simulink library "mech_stewart_control_deriv"  (Simulink 7.1)
values from neighbouring files (symbols this model uses):
  A = 100*freq    (= 314.159265359)    [mech_stewart_studies_setup.m]
libraries: mech_stewart_control_deriv x1
settings Model: Creator=batserve  LastModifiedBy=batserve  ExtModeAutoUpdateStatusClock=off

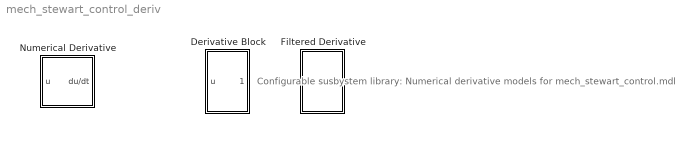
== system mech_stewart_control_deriv ==
  note: Configurable susbystem library:
      | Numerical derivative models for
      | mech_stewart_control.mdl
  Derivative Block : Subsystem
  Filtered Derivative : Subsystem
  "Numerical Derivative " : Subsystem  BlockChoice=Derivative Block
      settings: TemplateBlock=self  MemberBlocks=Derivative Block,Filtered Derivative

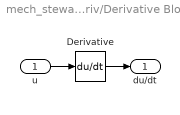
== system mech_stewart_control_deriv/Derivative Block ==
  u : Inport  OutDataType=sfix(16)  OutScaling=2^0
  Derivative : Derivative
  du/dt : Outport  OutDataType=sfix(16)  OutScaling=2^0
  wires:
  Derivative/1 -> du/dt/1
  u/1 -> Derivative/1

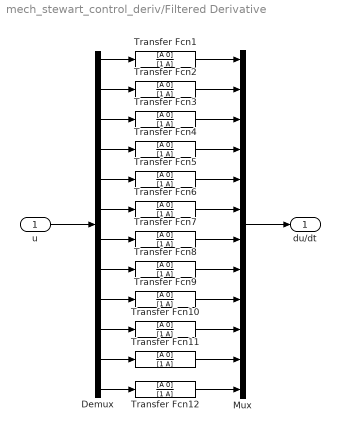
== system mech_stewart_control_deriv/Filtered Derivative ==
  u : Inport  OutDataType=sfix(16)  OutScaling=2^0
  Demux : Demux  Outputs=12
  Mux : Mux  Inputs=12
  Transfer Fcn{1..12} (12 alike) : TransferFcn  Numerator=[A 0]  Denominator=[1 A]
  du/dt : Outport  OutDataType=sfix(16)  OutScaling=2^0
  wires:
  Mux/1 -> du/dt/1
  u/1 -> Demux/1
  Demux/1 -> Transfer Fcn1/1
  Transfer Fcn1/1 -> Mux/1
  Demux/2 -> Transfer Fcn2/1
  Transfer Fcn2/1 -> Mux/2
  Demux/3 -> Transfer Fcn3/1
  Transfer Fcn3/1 -> Mux/3
  Demux/4 -> Transfer Fcn4/1
  Transfer Fcn4/1 -> Mux/4
  Demux/5 -> Transfer Fcn5/1
  Transfer Fcn5/1 -> Mux/5
  Demux/6 -> Transfer Fcn6/1
  Transfer Fcn6/1 -> Mux/6
  Demux/7 -> Transfer Fcn7/1
  Transfer Fcn7/1 -> Mux/7
  Demux/8 -> Transfer Fcn8/1
  Transfer Fcn8/1 -> Mux/8
  Demux/9 -> Transfer Fcn9/1
  Transfer Fcn9/1 -> Mux/9
  Demux/10 -> Transfer Fcn10/1
  Transfer Fcn10/1 -> Mux/10
  Demux/11 -> Transfer Fcn11/1
  Transfer Fcn11/1 -> Mux/11
  Demux/12 -> Transfer Fcn12/1
  Transfer Fcn12/1 -> Mux/12

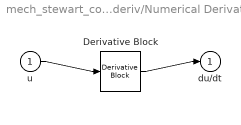
== system mech_stewart_control_deriv/Numerical Derivative  ==
  u : Inport  OutDataType=sfix(16)  OutScaling=2^0
  Derivative Block : mech_stewart_control_deriv/Derivative Block  SystemSampleTime=-1
  du/dt : Outport  OutDataType=sfix(16)  OutScaling=2^0
  wires:
  u/1 -> Derivative Block/1
  Derivative Block/1 -> du/dt/1
